simulink model "regulator_PI_simulink"  (R2025b)
settings: Solver=VariableStepAuto  StartTime=0.0  StopTime=150  RelTol=1e-3
values from neighbouring files (symbols this model uses):
  I_simulink = Kp_Bode/Ti_Bode    [Regulator_PI.m]
  K_oscylacje = ZapasWzmocnieniaBezwymiarowy_bode    [Regulator_PI.m]
  Kp_Bode = 0.45*K_oscylacje    [Regulator_PI.m]
  L1 = [3]    [Regulator_PI.m]
  L22 = [Kp_Bode*Ti_Bode Kp_Bode]    [Regulator_PI.m]
  L33 = [Kp_Tau_T*Ti_Tau_T Kp_Tau_T]    [Regulator_PI.m]
  L55 = [Kp_optymalizacja*Ti_stalaCzasowa Kp_optymalizacja]    [Regulator_PI.m]
  M1 = conv(m4,m5)    [Regulator_PI.m]
  M22 = [Ti_Bode 0]    [Regulator_PI.m]
  M33 = [Ti_Tau_T 0]    [Regulator_PI.m]
  M55 = [Ti_stalaCzasowa 0]    [Regulator_PI.m]
  Sample_time = 0.1    [Regulator_PI.m]
  Ti_Bode = T_oscylacje/(1.2)    [Regulator_PI.m]
libraries: slpidlib x1
settings Model: LastModifiedBy=mefir

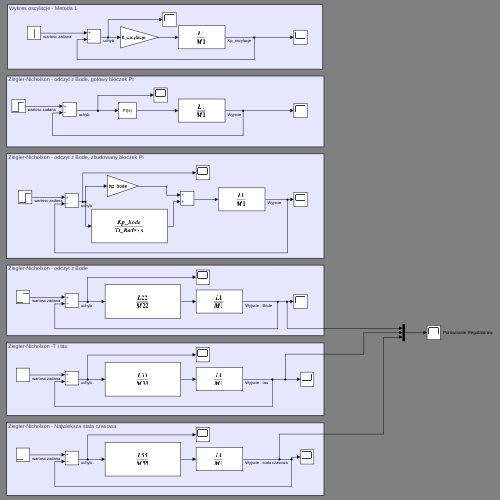
[thumbnail: Simulink's stored preview of the top-level diagram]
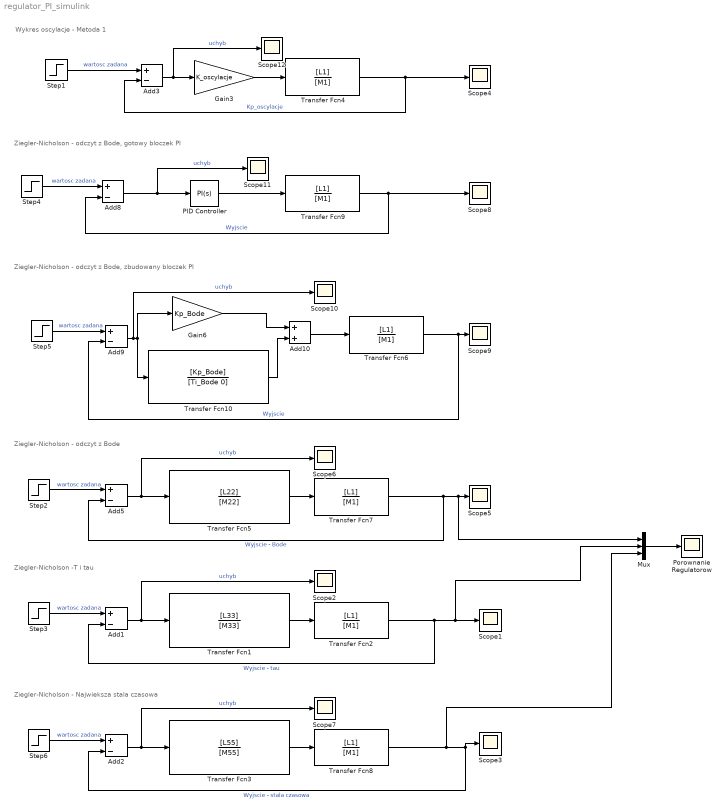
== system regulator_PI_simulink ==
  note: Ziegler-Nicholson - odczyt z Bode, zbudowany bloczek PI
  note: Ziegler-Nicholson - odczyt z Bode, gotowy bloczek PI
  note: Wykres oscylacje - Metoda 1
  note: Ziegler-Nicholson - odczyt z Bode
  note: Ziegler-Nicholson -T i tau
  note: Ziegler-Nicholson - Najwieksza stala czasowa
  Add{1..3,5,8..9} (6 alike) : Sum  Inputs=+-
  Add10 : Sum
  Gain3 : Gain  Gain=K_oscylacje
  Gain6 : Gain  Gain=Kp_Bode
  Mux : Mux  Inputs=3
  PID Controller : slpidlib/PID Controller  Controller=PI  Form=Parallel  TimeDomain=Continuous-time  UseExternalTs=off  SampleTime=-1  IntegratorMethod=Forward Euler  FilterMethod=Forward Euler  ControllerParametersSource=internal  P=Kp_Bode  I=I_simulink  UseKiTs=off  D=0  UseExternalDerivativeSource=off  N=100  UseFilter=on  TunerSelectOption=Transfer Function Based (PID Tuner App)  InitialConditionSource=internal  InitialConditionForIntegrator=0  InitialConditionForFilter=0  DifferentiatorICPrevScaledInput=0  ExternalReset=none  TrackingMode=off  Kt=1  LimitOutput=off  SatLimitsSource=internal  UpperSaturationLimit=inf  LowerSaturationLimit=-inf  LinearizeAsGain=on  AntiWindupMode=none  Kb=1  LimitIntegrator=off  UpperIntegratorSaturationLimit=inf  LowerIntegratorSaturationLimit=-inf  POutMin=[]  POutMax=[]  IOutMin=[]  IOutMax=[]  DOutMin=[]  DOutMax=[]  NOutMin=[]  NOutMax=[]  SumOutMin=[]  SumOutMax=[]  SaturationOutMin=[]  SaturationOutMax=[]  PParamMin=[]  PParamMax=[]  IParamMin=[]  IParamMax=[]  DParamMin=[]  DParamMax=[]  NParamMin=[]  NParamMax=[]  KbParamMin=[]  KbParamMax=[]  KtParamMin=[]  KtParamMax=[]  KbOutMin=[]  KbOutMax=[]  KtOutMin=[]  KtOutMax=[]  IntegratorOutMin=[]  IntegratorOutMax=[]  FilterOutMin=[]  FilterOutMax=[]  SumI1OutMin=[]  SumI1OutMax=[]  SumI2OutMin=[]  SumI2OutMax=[]  SumI3OutMin=[]  SumI3OutMax=[]  SumI4OutMin=[]  SumI4OutMax=[]  SumDOutMin=[]  SumDOutMax=[]  DifferentiatorOutMin=[]  DifferentiatorOutMax=[]  FilterDiffOutCoefMin=[]  FilterDiffOutCoefMax=[]  ReciprocalOutMin=[]  ReciprocalOutMax=[]  SumDenOutMin=[]  SumDenOutMax=[]  SumNumOutMin=[]  SumNumOutMax=[]  DivideOutMin=[]  DivideOutMax=[]  UdiffTsProdOutMin=[]  UdiffTsProdOutMax=[]  NTsProdOutMin=[]  NTsProdOutMax=[]  UintegralTsProdOutMin=[]  UintegralTsProdOutMax=[]  UngainTsProdOutMin=[]  UngainTsProdOutMax=[]  ClampingZeroOutDataTypeStr=Inherit: Inherit via back propagation  ClampingZeroOutMin=[]  ClampingZeroOutMax=[]  FilterDenConstantOutDataTypeStr=Inherit: Inherit via back propagation  FilterDenConstantOutMin=[]  FilterDenConstantOutMax=[]  PCopyOutDataTypeStr=Inherit: Inherit via back propagation  PCopyOutMin=[]  PCopyOutMax=[]  NCopyOutDataTypeStr=Inherit: Inherit via back propagation  NCopyOutMin=[]  NCopyOutMax=[]  IntegratorContinuousStateAttributes=''  IntegratorStateMustResolveToSignalObject=off  IntegratorRTWStateStorageClass=Auto  FilterContinuousStateAttributes=''  FilterStateMustResolveToSignalObject=off  FilterRTWStateStorageClass=Auto  ParallelPVariant=InternalParameters  IdealPVariant=Disabled  IVariant=InternalParameters  DVariant=Disabled  IntegratorVariant=Continuous  SatVariant=Disabled  AWVariant=Passthrough  PCopyVariant=Disabled  TRVariant=Disabled  FdbkBlocksVariant=Forward  IdealPFdbkVariant=Disabled  SatFdbkVariant=Disabled  DerivativeFilterVariant=Disabled  NVariant=Disabled  NCopyVariant=Disabled_SignalSpec  FilterICVariant=Disabled  IntegratorICVariant=InternalICs  ExternalResetVariant=Disabled  TRSumVariant=Passthrough  SumFdbkVariant=Disabled  SumVariant=Sum_PI  TsampFilterVariant=InternalTs  TsampNgainVariant=Passthrough  TsampIntegralVariant=Disabled_SignalSpec  ExternalSaturationOutDataTypeStr=Inherit: Same as second input  DerivativeSourceVariant=Disabled  PreIntVariant=InternalPreInt
  Porownanie Regulatorow : Scope
      settings: ActiveDisplayYMinimum=-1.1491294790076525  ActiveDisplayYMaximum=2.6607619283357895  DataLoggingVariableName=ScopeData7
  Scope{1..12} (12 alike) : Scope
      Scope1 settings: ActiveDisplayYMinimum=-1.1491294790076525  ActiveDisplayYMaximum=2.6607619283357895
      Scope10 settings: ActiveDisplayYMinimum=-1.1491294790076525  ActiveDisplayYMaximum=2.6607619283357895  DataLoggingVariableName=ScopeData10
      Scope11 settings: ActiveDisplayYMinimum=-1.1491294790076525  ActiveDisplayYMaximum=2.6607619283357895  DataLoggingVariableName=ScopeData11
      Scope12 settings: ActiveDisplayYMinimum=-1.1491294790076525  ActiveDisplayYMaximum=2.6607619283357895  DataLoggingVariableName=ScopeData12
      Scope2 settings: ActiveDisplayYMinimum=-1.1491294790076525  ActiveDisplayYMaximum=2.6607619283357895
      Scope3 settings: ActiveDisplayYMinimum=-1.1491294790076525  ActiveDisplayYMaximum=2.6607619283357895  DataLoggingVariableName=ScopeData2
      Scope4 settings: ActiveDisplayYMinimum=-1.3587201859755582  ActiveDisplayYMaximum=2.9907675699860246  DataLoggingVariableName=ScopeData4
      Scope5 settings: ActiveDisplayYMinimum=-1.1491294790076525  ActiveDisplayYMaximum=2.6607619283357895  DataLoggingVariableName=ScopeData5
      Scope6 settings: ActiveDisplayYMinimum=-1.1491294790076525  ActiveDisplayYMaximum=2.6607619283357895  DataLoggingVariableName=ScopeData6
      Scope7 settings: ActiveDisplayYMinimum=-1.1491294790076525  ActiveDisplayYMaximum=2.6607619283357895  DataLoggingVariableName=ScopeData3
      Scope8 settings: ActiveDisplayYMinimum=-0.19718197920927938  ActiveDisplayYMaximum=1.774637812883515  DataLoggingVariableName=ScopeData8
      Scope9 settings: ActiveDisplayYMinimum=-1.1491294790076525  ActiveDisplayYMaximum=2.6607619283357895  DataLoggingVariableName=ScopeData9
  Step{1..6} (6 alike) : Step  Time=0  SampleTime=Sample_time
  Transfer Fcn1 : TransferFcn  Numerator=[L33]  Denominator=[M33]
  Transfer Fcn10 : TransferFcn  Numerator=[Kp_Bode]  Denominator=[Ti_Bode 0]
  Transfer Fcn{2,4,6..9} (6 alike) : TransferFcn  Numerator=[L1]  Denominator=[M1]
  Transfer Fcn3 : TransferFcn  Numerator=[L55]  Denominator=[M55]
  Transfer Fcn5 : TransferFcn  Numerator=[L22]  Denominator=[M22]
  wires:
  Step1/1 -> Add3/1  "wartosc zadana"
  Add3/1 -> Scope12/1, Gain3/1  "uchyb"
  Transfer Fcn4/1 -> Add3/2, Scope4/1  "Kp_oscylacje"
  Gain3/1 -> Transfer Fcn4/1
  Transfer Fcn9/1 -> Scope8/1, Add8/2  "Wyjscie"
  Step4/1 -> Add8/1  "wartosc zadana"
  PID Controller/1 -> Transfer Fcn9/1
  Add8/1 -> Scope11/1, PID Controller/1  "uchyb"
  Gain6/1 -> Add10/1
  Transfer Fcn6/1 -> Scope9/1, Add9/2  "Wyjscie"
  Transfer Fcn10/1 -> Add10/2
  Step5/1 -> Add9/1  "wartosc zadana"
  Add10/1 -> Transfer Fcn6/1
  Add9/1 -> Scope10/1, Transfer Fcn10/1, Gain6/1  "uchyb"
  Transfer Fcn7/1 -> Mux/1, Scope5/1, Add5/2  "Wyjscie - Bode"
  Step2/1 -> Add5/1  "wartosc zadana"
  Add5/1 -> Scope6/1, Transfer Fcn5/1  "uchyb"
  Transfer Fcn5/1 -> Transfer Fcn7/1
  Transfer Fcn1/1 -> Transfer Fcn2/1
  Add1/1 -> Scope2/1, Transfer Fcn1/1  "uchyb"
  Transfer Fcn2/1 -> Add1/2, Mux/2, Scope1/1  "Wyjscie - tau"
  Step3/1 -> Add1/1  "wartosc zadana"
  Transfer Fcn3/1 -> Transfer Fcn8/1
  Add2/1 -> Scope7/1, Transfer Fcn3/1  "uchyb"
  Transfer Fcn8/1 -> Mux/3, Add2/2, Scope3/1  "Wyjscie - stala czasowa"
  Step6/1 -> Add2/1  "wartosc zadana"
  Mux/1 -> Porownanie Regulatorow/1
